simulink model "ScienceStimHasomed_test"  (Simulink 8.0)
settings: Solver=FixedStepDiscrete  StartTime=0.0  StopTime=50  FixedStep=0.05  RelTol=1e-3
libraries: ScienceStimHasomed_Lib x1, rtsync_lib x1
settings Model: Creator=henrik  LastModifiedBy=Thomas Schauer
settings DataIOCC: SignalLoggingSaveFormat=ModelDataLogs
settings OptimizationCC: InitFltsAndDblsToZero=on
settings DebuggingCC: SaveWithParameterizedLinksMsg=none  SignalResolutionControl=TryResolveAllWithWarning  MultiTaskDSMMsg=warning  MultiTaskCondExecSysMsg=none  FcnCallInpInsideContextMsg=UseLocalSettings  StrictBusMsg=None
settings RTWCC: IncludeERTFirstTime=on
settings GRTTargetCC: TargetFcnLib=ansi_tfl_tmw.mat  CombineOutputUpdateFcns=off  GRTInterface=on

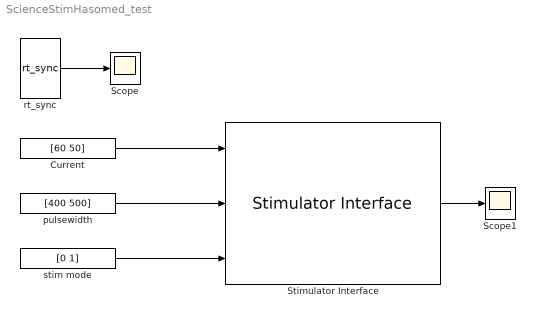
== system ScienceStimHasomed_test ==
  Current : Constant  Value=[60 50]
  Scope : Scope
      settings: YMin=0.05  YMax=0.05
  Scope1 : Scope
      settings: YMin=0  YMax=0.1
  Stimulator Interface : ScienceStimHasomed_Lib/Stimulator Interface  Ts=0.05  com_port=COM3  channelstim=[1 2]  tsone=0  tstwo=4  channellf=[]  nfactor=[]  outflag=on  dtflag=on
  pulsewidth : Constant  Value=[400 500]
  rt_sync : rtsync_lib/rt_sync  Ts=0.05  strict=off  outflag=on
  stim mode : Constant  Value=[0 1]
  wires:
  rt_sync/1 -> Scope/1
  Stimulator Interface/1 -> Scope1/1
  Current/1 -> Stimulator Interface/1
  pulsewidth/1 -> Stimulator Interface/2
  stim mode/1 -> Stimulator Interface/3
